simulink model "untitled"  (R2016a)
settings: Solver=ode4  StartTime=0.0  StopTime=5  FixedStep=0.001  RelTol=1e-3
settings Model: Creator=2083986g  LastModifiedBy=2083986g

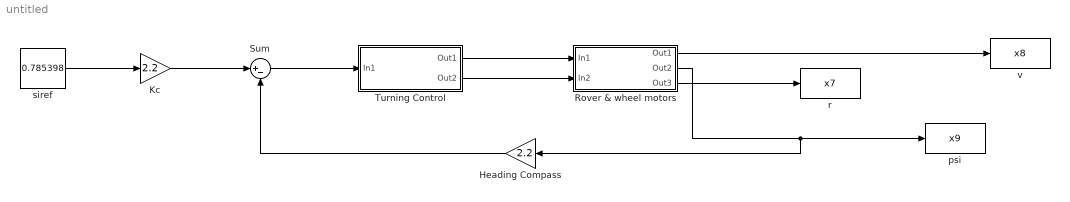
== system untitled ==
  Heading Compass : Gain  Gain=2.2
  Kc : Gain  Gain=2.2
  Rover & wheel motors : Subsystem
  Sum : Sum  Inputs=|+-
  Turning Control : Subsystem
  psi : ToWorkspace  VariableName=x9  SampleTime=-1
  r : ToWorkspace  VariableName=x7  SampleTime=-1
  siref : Constant  Value=0.785398
  v : ToWorkspace  VariableName=x8  SampleTime=-1
  wires:
  Kc/1 -> Sum/1
  Sum/1 -> Turning Control/1(In1)
  Turning Control/1(Out1) -> Rover & wheel motors/1(In1)
  Heading Compass/1 -> Sum/2
  Turning Control/2(Out2) -> Rover & wheel motors/2(In2)
  Rover & wheel motors/3(Out3) -> r/1
  Rover & wheel motors/2(Out2) -> Heading Compass/1, psi/1
  Rover & wheel motors/1(Out1) -> v/1
  siref/1 -> Kc/1

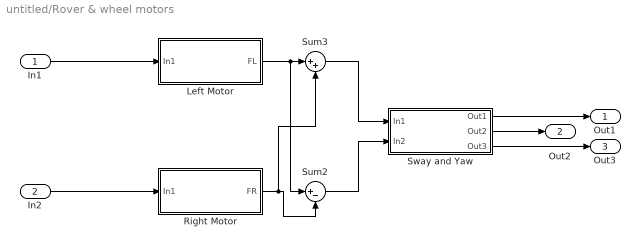
== system untitled/Rover & wheel motors ==
  In1 : Inport
  In2 : Inport  Port=2
  "Left Motor " : Subsystem
  Right Motor : Subsystem
  Sum2 : Sum  Inputs=|+-
  Sum3 : Sum  Inputs=|++
  "Sway and Yaw " : Subsystem
  Out1 : Outport
  Out2 : Outport  Port=2
  Out3 : Outport  Port=3
  wires:
  "Sway and Yaw "/1(Out1) -> Out1/1
  "Sway and Yaw "/3(Out3) -> Out3/1
  "Sway and Yaw "/2(Out2) -> Out2/1
  "Left Motor "/1(FL) -> Sum2/1, Sum3/1
  Right Motor/1(FR) -> Sum3/2, Sum2/2
  Sum3/1 -> "Sway and Yaw "/1(In1)
  Sum2/1 -> "Sway and Yaw "/2(In2)
  In2/1 -> Right Motor/1(In1)
  In1/1 -> "Left Motor "/1(In1)

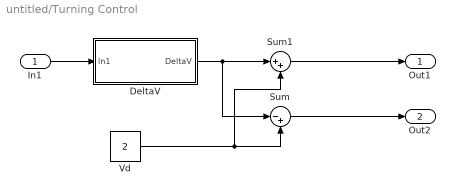
== system untitled/Turning Control ==
  In1 : Inport
  DeltaV : Subsystem
  Sum : Sum  Inputs=|-+
  Sum1 : Sum  Inputs=|++
  Vd : Constant  Value=2
  Out1 : Outport
  Out2 : Outport  Port=2
  wires:
  In1/1 -> DeltaV/1(ln1)
  Vd/1 -> Sum1/2, Sum/2
  Sum/1 -> Out2/1
  Sum1/1 -> Out1/1
  DeltaV/1(DeltaV) -> Sum/1, Sum1/1

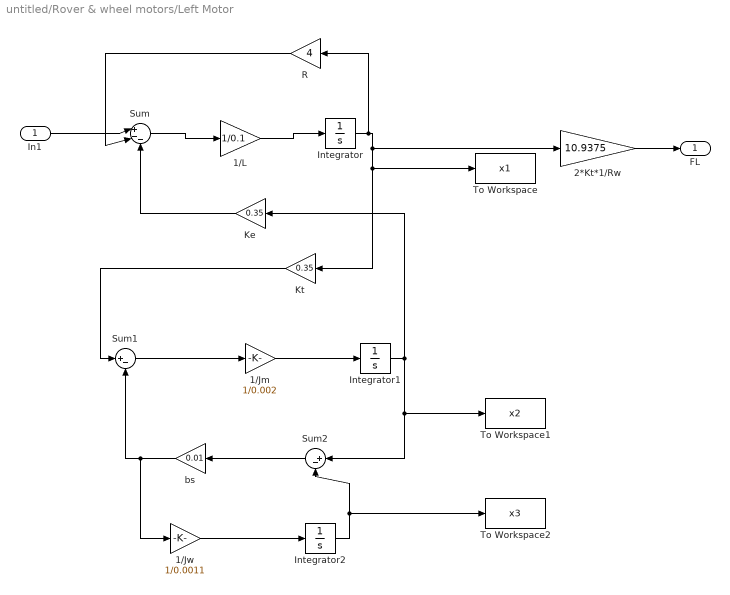
== system untitled/Rover & wheel motors/Left Motor  ==
  In1 : Inport
  1/Jm : Gain  Gain=1/0.002
  1/Jw : Gain  Gain=1/0.0011
  1/L : Gain  Gain=1/0.1
  2*Kt*1/Rw : Gain  Gain=10.9375
  Integrator : Integrator
  Integrator1 : Integrator
  Integrator2 : Integrator
  Ke : Gain  Gain=0.35
  Kt : Gain  Gain=0.35
  R : Gain  Gain=4
  Sum : Sum  Inputs=|+--
  Sum1 : Sum  Inputs=|+-
  Sum2 : Sum  Inputs=|+-
  To Workspace : ToWorkspace  VariableName=x1  SampleTime=-1
  To Workspace1 : ToWorkspace  VariableName=x2  SampleTime=-1
  To Workspace2 : ToWorkspace  VariableName=x3  SampleTime=-1
  bs : Gain  Gain=0.01
  FL : Outport
  wires:
  In1/1 -> Sum/1
  Sum/1 -> 1/L/1
  1/L/1 -> Integrator/1
  R/1 -> Sum/2
  Ke/1 -> Sum/3
  Kt/1 -> Sum1/1
  Sum1/1 -> 1/Jm/1
  1/Jm/1 -> Integrator1/1
  bs/1 -> 1/Jw/1, Sum1/2
  Sum2/1 -> bs/1
  Integrator1/1 -> Sum2/1, To Workspace1/1, Ke/1
  1/Jw/1 -> Integrator2/1
  Integrator2/1 -> To Workspace2/1, Sum2/2
  Integrator/1 -> R/1, Kt/1, To Workspace/1, 2*Kt*1/Rw/1
  2*Kt*1/Rw/1 -> FL/1

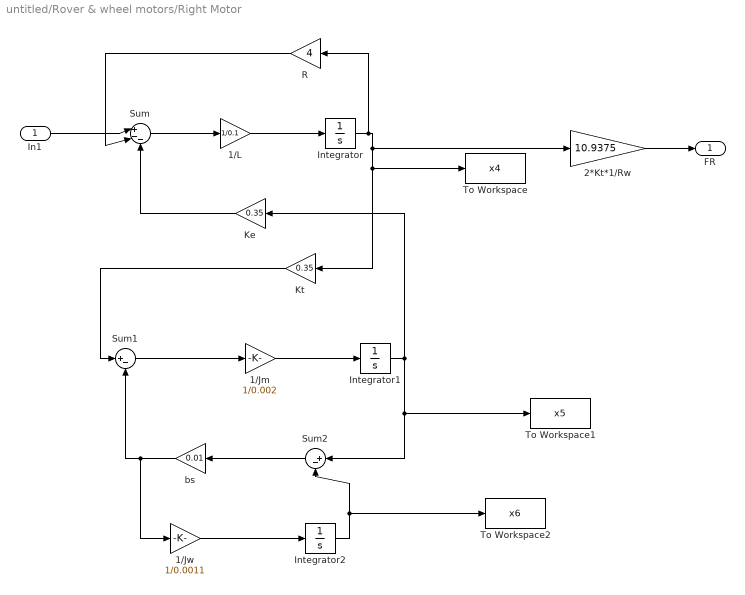
== system untitled/Rover & wheel motors/Right Motor ==
  In1 : Inport
  1/Jm : Gain  Gain=1/0.002
  1/Jw : Gain  Gain=1/0.0011
  1/L : Gain  Gain=1/0.1
  2*Kt*1/Rw : Gain  Gain=10.9375
  Integrator : Integrator
  Integrator1 : Integrator
  Integrator2 : Integrator
  Ke : Gain  Gain=0.35
  Kt : Gain  Gain=0.35
  R : Gain  Gain=4
  Sum : Sum  Inputs=|+--
  Sum1 : Sum  Inputs=|+-
  Sum2 : Sum  Inputs=|+-
  To Workspace : ToWorkspace  VariableName=x4  SampleTime=-1
  To Workspace1 : ToWorkspace  VariableName=x5  SampleTime=-1
  To Workspace2 : ToWorkspace  VariableName=x6  SampleTime=-1
  bs : Gain  Gain=0.01
  FR : Outport
  wires:
  In1/1 -> Sum/1
  Sum/1 -> 1/L/1
  1/L/1 -> Integrator/1
  R/1 -> Sum/2
  Ke/1 -> Sum/3
  Kt/1 -> Sum1/1
  Sum1/1 -> 1/Jm/1
  1/Jm/1 -> Integrator1/1
  bs/1 -> 1/Jw/1, Sum1/2
  Sum2/1 -> bs/1
  Integrator1/1 -> Sum2/1, To Workspace1/1, Ke/1
  1/Jw/1 -> Integrator2/1
  Integrator2/1 -> To Workspace2/1, Sum2/2
  Integrator/1 -> R/1, Kt/1, To Workspace/1, 2*Kt*1/Rw/1
  2*Kt*1/Rw/1 -> FR/1

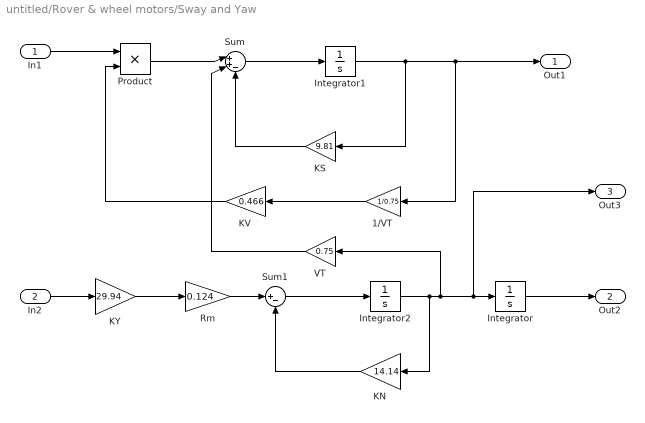
== system untitled/Rover & wheel motors/Sway and Yaw  ==
  In1 : Inport
  In2 : Inport  Port=2
  1/VT : Gain  Gain=1/0.75
  Integrator : Integrator
  Integrator1 : Integrator
  Integrator2 : Integrator
  KN : Gain  Gain=14.14
  KS : Gain  Gain=9.81
  KV : Gain  Gain=0.466
  KY : Gain  Gain=29.94
  Product : Product
  Rm : Gain  Gain=0.124
  Sum : Sum  Inputs=|++-
  Sum1 : Sum  Inputs=|+-
  VT : Gain  Gain=0.75
  Out1 : Outport
  Out2 : Outport  Port=2
  Out3 : Outport  Port=3
  wires:
  In1/1 -> Product/1
  Product/1 -> Sum/1
  Sum/1 -> Integrator1/1
  Integrator1/1 -> KS/1, 1/VT/1, Out1/1
  KS/1 -> Sum/3
  1/VT/1 -> KV/1
  In2/1 -> KY/1
  KY/1 -> Rm/1
  Rm/1 -> Sum1/1
  KN/1 -> Sum1/2
  Sum1/1 -> Integrator2/1
  Integrator2/1 -> KN/1, VT/1, Out3/1, Integrator/1
  Integrator/1 -> Out2/1
  KV/1 -> Product/2
  VT/1 -> Sum/2

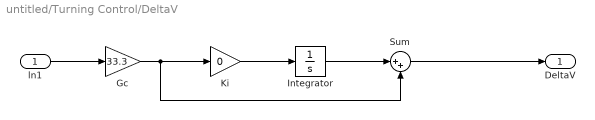
== system untitled/Turning Control/DeltaV ==
  ln1 : Inport
  Gc : Gain  Gain=33.3
  Integrator : Integrator
  Ki : Gain  Gain=0
  Sum : Sum  Inputs=|++
  DeltaV : Outport
  wires:
  ln1/1 -> Gc/1
  Gc/1 -> Sum/2, Ki/1
  Ki/1 -> Integrator/1
  Integrator/1 -> Sum/1
  Sum/1 -> DeltaV/1
